simulink subsystem "Main_Kalman_1D_Augmented_Block"  (R2024a)
settings: Solver=VariableStepAuto  StartTime=0.0  StopTime=10.0  RelTol=1e-3
undefined symbols (not defined in the file): Ad_aug, Bd_aug, Cd_aug, Discrete, R_aug_kf, Time
libraries: ctrlSharedLib x1
settings Model: Creator=Peter  LastModifiedBy=Peter

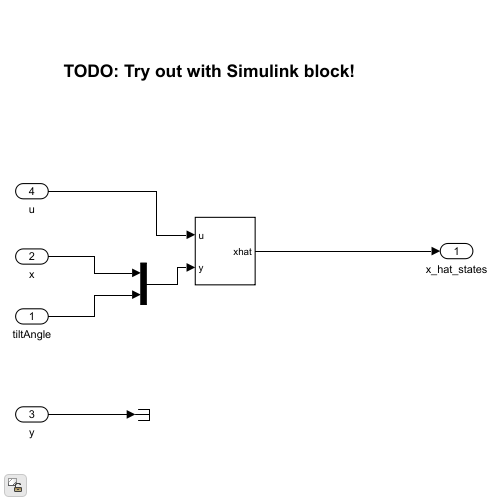
[thumbnail: Simulink's stored preview of the top-level diagram]
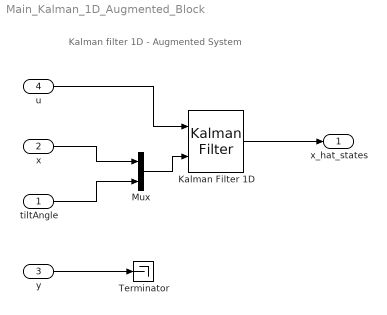
== system Main_Kalman_1D_Augmented_Block ==
  note: Kalman filter 1D - Augmented System
  tiltAngle : Inport  OutDataTypeStr=single
  x : Inport  Port=2  OutDataTypeStr=single
  y : Inport  Port=3  OutDataTypeStr=single
  u : Inport  Port=4  OutDataTypeStr=single
  Kalman Filter 1D : ctrlSharedLib/Kalman Filter  TimeDomain=Discrete-Time  UseCurrentEstimator=on  ModelSource=Individual A, B, C, D matrices  ModelSourceVariable=ss(0.95,1,1,0,1)  A=Ad_aug  B=Bd_aug  C=Cd_aug  D=0  NumberOfStates=1  NumberOfInputs=1  NumberOfOutputs=1  InitialEstimateSource=Dialog  X0=[0;0;0;0;0;0]  P0=10  UseK=off  UseGH=off  NumberOfProcessNoiseInputs=1  G=eye(6)  TimeInvariantG=on  H=[1 0 0 0 0 0;0 0 1 0 0 0]  TimeInvariantH=on  Q=Q_aug_kf  TimeInvariantQ=on  R=R_aug_kf  TimeInvariantR=on  N=0  TimeInvariantN=on  AddInputPort=on  AddEnablePort=off  OutputEstimatedY=off  OutputP=off  Ts=-1
  Mux : Mux  Inputs=2
  Terminator : Terminator
  x_hat_states : Outport  OutDataTypeStr=single
  wires:
  u/1 -> Kalman Filter 1D/1
  Kalman Filter 1D/1 -> x_hat_states/1
  x/1 -> Mux/1
  tiltAngle/1 -> Mux/2
  y/1 -> Terminator/1
  Mux/1 -> Kalman Filter 1D/2
